simulink model "ai_guidance_depth_hz50_200917"  (R2021a)
settings: Solver=FixedStepDiscrete  StartTime=0.0  StopTime=inf  FixedStep=0.02  RelTol=1e-3  EnableMultiTasking=on
model workspace (MAT data in the model file):
  SL_ROS_VariableLengthArrays_MaxSizes.CommonInfo.ArrayTruncateAction = 'EmitWarning'
  SL_ROS_VariableLengthArrays_MaxSizes.MsgTypeMap = containers.Map
  SL_ROS_VariableLengthArrays_MaxSizes.MsgTypeMap.serialization.keys = {'sensor_msgs/LaserScan', 'std_msgs/Float32MultiArray', 'std_msgs/Float64MultiArray'}
  SL_ROS_VariableLengthArrays_MaxSizes.MsgTypeMap.serialization.values{1}(1).PropertyName = 'Intensities'
  SL_ROS_VariableLengthArrays_MaxSizes.MsgTypeMap.serialization.values{1}(1).DataType = 'single'
  SL_ROS_VariableLengthArrays_MaxSizes.MsgTypeMap.serialization.values{1}(1).MaxLength = 360
  SL_ROS_VariableLengthArrays_MaxSizes.MsgTypeMap.serialization.values{1}(2).PropertyName = 'Ranges'
  SL_ROS_VariableLengthArrays_MaxSizes.MsgTypeMap.serialization.values{1}(2).DataType = 'single'
  SL_ROS_VariableLengthArrays_MaxSizes.MsgTypeMap.serialization.values{1}(2).MaxLength = 360
  SL_ROS_VariableLengthArrays_MaxSizes.MsgTypeMap.serialization.values{2}.PropertyName = 'Data'
  SL_ROS_VariableLengthArrays_MaxSizes.MsgTypeMap.serialization.values{2}.DataType = 'single'
  SL_ROS_VariableLengthArrays_MaxSizes.MsgTypeMap.serialization.values{2}.MaxLength = 512
  SL_ROS_VariableLengthArrays_MaxSizes.MsgTypeMap.serialization.values{3}.PropertyName = 'Data'
  SL_ROS_VariableLengthArrays_MaxSizes.MsgTypeMap.serialization.values{3}.DataType = 'double'
  SL_ROS_VariableLengthArrays_MaxSizes.MsgTypeMap.serialization.values{3}.MaxLength = 360
  SL_ROS_VariableLengthArrays_MaxSizes.MsgTypeMap.serialization.uniformity = 0
  SL_ROS_VariableLengthArrays_MaxSizes.MsgTypeMap.serialization.keyType = 'char'
  SL_ROS_VariableLengthArrays_MaxSizes.MsgTypeMap.serialization.valueType = 'any'
undefined symbols (not defined in the file): Pose
libraries: robotlib x6, sharedtransform x1
settings Model: Creator=USER  LastModifiedBy=note
settings SolverCC: AlgebraicLoopSolver=TrustRegion
settings DataIOCC: ReturnWorkspaceOutputs=off
settings OptimizationCC: EnhancedBackFolding=on  PassReuseOutputArgsAs=Individual arguments  MaxStackSize=64  OptimizeBlockOrder=speed  DifferentSizesBufferReuse=on  OptimizationCustomize=off  EfficientTunableParamExpr=on
settings DebuggingCC: ParameterTunabilityLossMsg=error  PregeneratedLibrarySubsystemCodeDiagnostic=none  SFMachineParentedDataDiag=warning  ArithmeticOperatorsInVariantConditions=warning
settings HardwareCC: ProdBitPerPointer=32  ProdBitPerSizeT=32  ProdBitPerPtrDiffT=32  ProdLargestAtomicFloat=None  ProdIntDivRoundTo=Undefined  ProdEndianess=Unspecified  ProdWordSize=32  ProdHWDeviceType=Generic->Unspecified (assume 32-bit Generic)
settings SFSimCC: SimUseLocalCustomCode=off  MATLABDynamicMemAlloc=off  CustomCodeUndefinedFunction=UseInterfaceOnly  SimTargetLang=C++
settings RTWCC: SystemTargetFile=ert.tlc  HardwareBoard=Robot Operating System (ROS)  TLCOptions="-aInlineSetEventsForThisBaseRateFcn=TLC_FALSE -aSuppressMultiTaskScheduler=TLC_FALSE  -aRateBasedStepFcn=0"  TemplateMakefile=ert_default_tmf  GenerateReport=on  RTWUseLocalCustomCode=off  Toolchain=Catkin  BuildConfiguration=Faster Runs  IncludeHyperlinkInReport=on  LaunchReport=on  TargetLang=C++  GenerateTraceInfo=on  GenerateTraceReport=on  GenerateTraceReportSl=on  GenerateTraceReportSf=on  GenerateTraceReportEml=on
settings CodeAppCC: ForceParamTrailComments=on  IgnoreCustomStorageClasses=off  OperatorAnnotations=on  SimulinkDataObjDesc=on  SFDataObjDesc=on  InsertBlockDesc=on
settings ERTTargetCC: SupportVariableSizeSignals=on

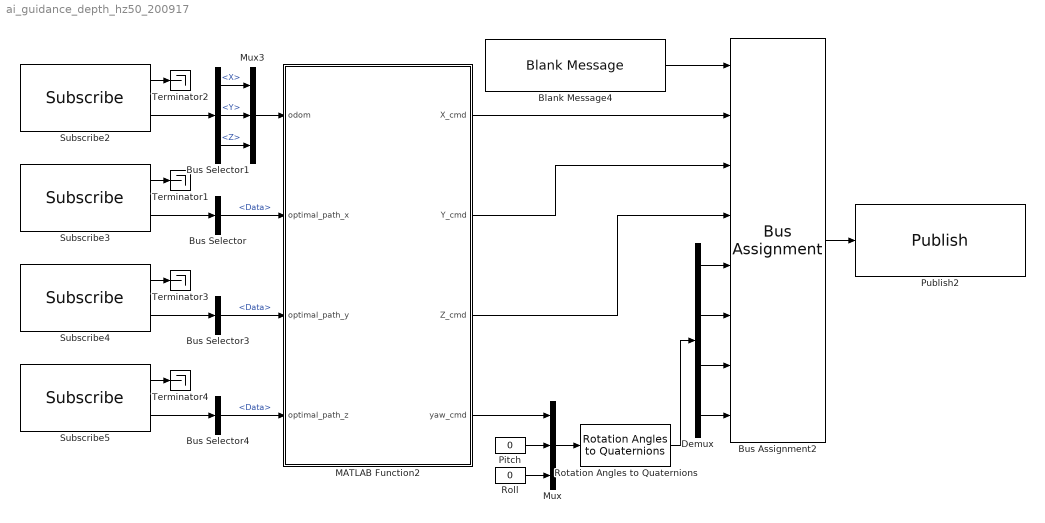
== system ai_guidance_depth_hz50_200917 ==
  " Roll" : Constant  Value=0  OutDataTypeStr=double  SampleTime=-1
  Blank Message4 : robotlib/Blank Message  messageClass=Message  entityType=geometry_msgs/PoseStamped  messageType=geometry_msgs/PoseStamped  SampleTime=-1  legacyBusStruct=off
  Bus Assignment2 : BusAssignment  AssignedSignals=Pose.Position.X,Pose.Position.Y,Pose.Position.Z,Pose.Orientation.W,Pose.Orientation.X,Pose.Orientation.Y,Pose.Orientation.Z
  Bus Selector : BusSelector  OutputSignals=Data
  Bus Selector1 : BusSelector  OutputSignals=Pose.Pose.Position.X,Pose.Pose.Position.Y,Pose.Pose.Position.Z
  Bus Selector3 : BusSelector  OutputSignals=Data
  Bus Selector4 : BusSelector  OutputSignals=Data
  Demux : Demux
  MATLAB Function2 : MATLAB Function  TreatAsAtomicUnit=on
  Mux : Mux  Inputs=3
  Mux3 : Mux  Inputs=3
  Pitch : Constant  Value=0  OutDataTypeStr=double  SampleTime=-1
  Publish2 : robotlib/Publish  topicSource=Select from ROS network  topic=/mavros/setpoint_position/local  messageType=geometry_msgs/PoseStamped  legacyBusStruct=off  messageQueueLength=1
  Rotation Angles to Quaternions : sharedtransform/Rotation Angles to Quaternions  rotationOrder=ZYX  aMode=aMode
      settings: SourceProductBaseCode=AE,PW,DR,MT,UV,VE
  Subscribe2 : robotlib/Subscribe  topicSource=Select from ROS network  topic=/rtabmap/odom  messageType=nav_msgs/Odometry  SampleTime=-1  legacyBusStruct=off  messageQueueLength=1
  Subscribe3 : robotlib/Subscribe  topicSource=Specify your own  topic=/optimal_path_x  messageType=std_msgs/Float32MultiArray  SampleTime=-1  legacyBusStruct=off  messageQueueLength=1
  Subscribe4 : robotlib/Subscribe  topicSource=Specify your own  topic=/optimal_path_y  messageType=std_msgs/Float32MultiArray  SampleTime=-1  legacyBusStruct=off  messageQueueLength=1
  Subscribe5 : robotlib/Subscribe  topicSource=Specify your own  topic=/optimal_path_z  messageType=std_msgs/Float32MultiArray  SampleTime=-1  legacyBusStruct=off  messageQueueLength=1
  Terminator{1..4} (4 alike) : Terminator
  wires:
  Subscribe3/2 -> Bus Selector/1
  Subscribe3/1 -> Terminator1/1
  Subscribe4/1 -> Terminator3/1
  Subscribe5/1 -> Terminator4/1
  Bus Assignment2/1 -> Publish2/1
  Subscribe4/2 -> Bus Selector3/1
  Subscribe5/2 -> Bus Selector4/1
  Bus Selector/1 -> MATLAB Function2/2(optimal_path_x)  "<Data>"
  Bus Selector3/1 -> MATLAB Function2/3(optimal_path_y)  "<Data>"
  Bus Selector4/1 -> MATLAB Function2/4(optimal_path_z)  "<Data>"
  Blank Message4/1 -> Bus Assignment2/1
  MATLAB Function2/1(X_cmd) -> Bus Assignment2/2
  MATLAB Function2/2(Y_cmd) -> Bus Assignment2/3
  MATLAB Function2/3(Z_cmd) -> Bus Assignment2/4
  MATLAB Function2/4(yaw_cmd) -> Mux/1
  Mux/1 -> Rotation Angles to Quaternions/1
  Pitch/1 -> Mux/2
  " Roll"/1 -> Mux/3
  Rotation Angles to Quaternions/1 -> Demux/1
  Demux/1 -> Bus Assignment2/5
  Demux/2 -> Bus Assignment2/6
  Demux/3 -> Bus Assignment2/7
  Demux/4 -> Bus Assignment2/8
  Mux3/1 -> MATLAB Function2/1(odom)
  Bus Selector1/1 -> Mux3/1  "<X>"
  Subscribe2/1 -> Terminator2/1
  Bus Selector1/2 -> Mux3/2  "<Y>"
  Subscribe2/2 -> Bus Selector1/1
  Bus Selector1/3 -> Mux3/3  "<Z>"

== matlab function ai_guidance_depth_hz50_200917/MATLAB Function2 ==
  data: X_cmd output; Y_cmd output; odom input; Z_cmd output; optimal_path_x input size=[512 1]; optimal_path_y input size=[512 1]; optimal_path_z input size=[512 1]; yaw_cmd output
function [X_cmd,Y_cmd,Z_cmd,yaw_cmd] = fcn(odom,optimal_path_x,optimal_path_y,optimal_path_z)

persistent yaw_mem yaw_inc hz_20

if isempty(yaw_mem)
   yaw_mem = 0;
   yaw_inc = 0;
   hz_20 = 0;
end

hz_20 = hz_20 + 1;

path_length = length(optimal_path_x);
K = inf(path_length,1);
optimal_path_norm = inf(path_length,3);

% optimal_path_x_temp = optimal_path_x.Data';
% optimal_path_y_temp = optimal_path_y.Data';

optimal_path_norm(:,1) = single(optimal_path_x - odom(1));
optimal_path_norm(:,2) = single(optimal_path_y - odom(2));
optimal_path_norm(:,3) = single(optimal_path_z - odom(3));

% optimal_path = [optimal_path_x' optimal_path_y'];
% optimal_path_norm = optimal_path - [odom(1) odom(2)];

for i=1:path_length
    K(i) = norm(optimal_path_norm(i,:));
end

[~,m] = min(K);

% Z_cmd = optimal_path_z(m);
if m >= 512
    m = 511;
end

% Z_cmd = double(optimal_path_z(m+1) + APF_vector(3));         % prediction
% X_cmd = double(optimal_path_x(m+1) + APF_vector(1));
% Y_cmd = double(optimal_path_y(m+1) + APF_vector(2));

Z_cmd = double(optimal_path_z(m+1));         % prediction
X_cmd = double(optimal_path_x(m+1));
Y_cmd = double(optimal_path_y(m+1));

if m <= 509
%     yaw_vector1 = [optimal_path_x(m+1)-odom(1) optimal_path_y(m+1)-odom(2)] / norm([optimal_path_x(m+1)-odom(1) optimal_path_y(m+1)-odom(2)]);
%     yaw_vector2 = [optimal_path_x(m+2)-odom(1) optimal_path_y(m+2)-odom(2)] / norm([optimal_path_x(m+2)-odom(1) optimal_path_y(m+2)-odom(2)]);
%     yaw_vector3 = [optimal_path_x(m+3)-odom(1) optimal_path_y(m+3)-odom(2)] / norm([optimal_path_x(m+3)-odom(1) optimal_path_y(m+3)-odom(2)]);
    yaw_vector1 = [optimal_path_x(m+1)-odom(1) optimal_path_y(m+1)-odom(2)];
    yaw_vector2 = [optimal_path_x(m+2)-odom(1) optimal_path_y(m+2)-odom(2)];
    yaw_vector3 = [optimal_path_x(m+3)-odom(1) optimal_path_y(m+3)-odom(2)];
    yaw_vector = yaw_vector1 + yaw_vector2 + yaw_vector3;
    if norm(yaw_vector3) <= 0.4
        yaw_cmd = 0;
    else
        yaw_cmd = double( atan2(yaw_vector(2),yaw_vector(1)) );
    end
    yaw_mem = yaw_cmd;
    yaw_inc = 0;
%     yaw_cmd = double( ( atan2(optimal_path_y(m+1)-odom(2),optimal_path_x(m+1)-odom(1)) + atan2(optimal_path_y(m+2)-odom(2),optimal_path_x(m+2)-odom(1)) + atan2(optimal_path_y(m+3)-odom(2),optimal_path_x(m+3)-odom(1)) ) / 3 );
else
    yaw_cmd = yaw_mem + deg2rad(yaw_inc);
end

if hz_20 == 80           
    hz_20 = 0;
    if m == 512
%         yaw_inc = yaw_inc + 30;        % 4초마다 30도 돌려서 관찰 
        yaw_inc = yaw_inc + 0;        
    end
end


if odom(1) == 0 && odom(2) == 0 && odom(3) == 0
    Z_cmd = nan(1,1);
    X_cmd = nan(1,1);
    Y_cmd = nan(1,1);
end
    
% yaw_cmd = 0;

end
